simulink model "BodeConSimulink_perdidas"  (R2021b)
settings: Solver=ode23t  StartTime=0.0  StopTime=50e-3  RelTol=1e-3
values from neighbouring files (symbols this model uses):
  amp_bode = amp_bode*0.5    (= 0.003)    [BodeMatlab.m]
  Duty = 0.5    [BodeMatlab.m]
  freq_bode = frec(k)    [BodeMatlab.m]
  sampling = 0.1e-6    (= 1e-07)    [BodeMatlab.m]
libraries: fl_lib x8, nesl_utility x3
settings Model: Creator=PC  LastModifiedBy=PC

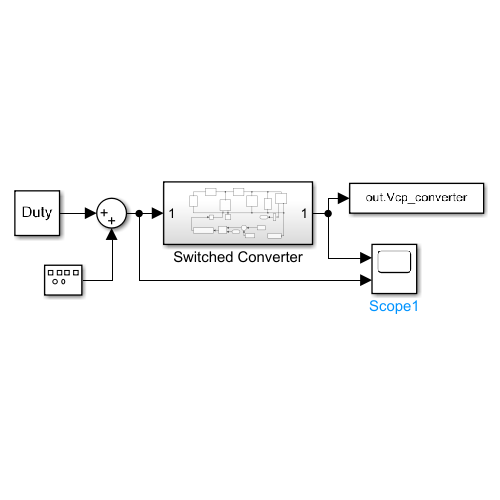
[thumbnail: Simulink's stored preview of the top-level diagram]
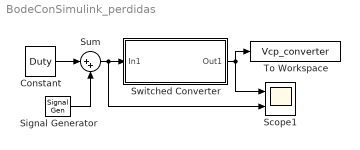
== system BodeConSimulink_perdidas ==
  " Switched Converter " : Subsystem
  Constant : Constant  Value=Duty  VectorParams1D=off  SampleTime=sampling
  Scope1 : Scope  NumInputPorts=2
  Signal Generator : SignalGenerator  Amplitude=amp_bode  Frequency=freq_bode
  Sum : Sum  Inputs=|++
  To Workspace : ToWorkspace  VariableName=Vcp_converter  SaveFormat=Structure With Time  SampleTime=-1
  wires:
  " Switched Converter "/1(Out1) -> Scope1/1, To Workspace/1
  Constant/1 -> Sum/1
  Sum/1 -> Scope1/2, " Switched Converter "/1(In1)
  Signal Generator/1 -> Sum/2

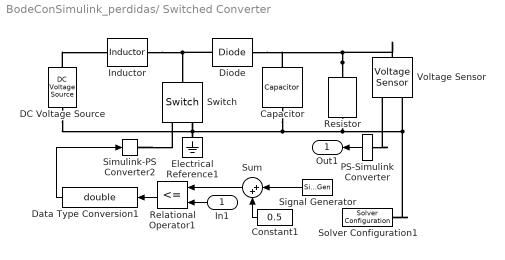
== system BodeConSimulink_perdidas/ Switched Converter  ==
  In1 : Inport
  Capacitor : fl_lib/Electrical/Electrical Elements/Capacitor  c=23 uF  r=20e-3 Ohm  g=0 1/Ohm  i_specify=off  i_priority=None  i=0 A  i_nominal_specify=off  i_nominal_unit=A  i_nominal_value=1  v_specify=off  v_priority=None  v=0 V  v_nominal_specify=off  v_nominal_unit=V  v_nominal_value=1  vc_specify=off  vc_priority=High  vc=0 V  vc_nominal_specify=off  vc_nominal_unit=V  vc_nominal_value=1
  Constant1 : Constant  Value=0.5  SampleTime=sampling
  DC Voltage Source : fl_lib/Electrical/Electrical Sources/DC Voltage Source  v0=12 V
  Data Type Conversion1 : DataTypeConversion  OutDataTypeStr=double
  Diode : fl_lib/Electrical/Electrical Elements/Diode  Vf=1.5 V  Ron=0.72 Ohm  Goff=1e-8 1/Ohm  i_specify=off  i_priority=None  i=0 A  i_nominal_specify=off  i_nominal_unit=A  i_nominal_value=1  v_specify=off  v_priority=None  v=0 V  v_nominal_specify=off  v_nominal_unit=V  v_nominal_value=1
  Electrical Reference1 : fl_lib/Electrical/Electrical Elements/Electrical Reference
  Inductor : fl_lib/Electrical/Electrical Elements/Inductor  l=130.2 uH  r=130e-3 Ohm  g=0 1/Ohm  i_specify=off  i_priority=None  i=0 A  i_nominal_specify=off  i_nominal_unit=A  i_nominal_value=1  v_specify=off  v_priority=None  v=0 V  v_nominal_specify=off  v_nominal_unit=V  v_nominal_value=1  i_L_specify=off  i_L_priority=High  i_L=0 A  i_L_nominal_specify=off  i_L_nominal_unit=A  i_L_nominal_value=1
  PS-Simulink Converter : nesl_utility/PS-Simulink Converter  PhysicalDomain=network_engine_domain  SubClassName=ps_output  LeftPortType=input  RightPortType=output  PseudoPeriodic=off  Frequencies=[]  Unit=inherit  AffineConversion=off
      settings: SourceProductBaseCode=PW,SS
  Relational Operator1 : RelationalOperator  Operator=<=  OutDataTypeStr=boolean  RndMeth=Simplest
  Resistor : fl_lib/Electrical/Electrical Elements/Resistor  R=50 Ohm  i_specify=off  i_priority=None  i=0 A  i_nominal_specify=off  i_nominal_unit=A  i_nominal_value=1  v_specify=off  v_priority=None  v=0 V  v_nominal_specify=off  v_nominal_unit=V  v_nominal_value=1
  Signal Generator : SignalGenerator  WaveForm=sawtooth  Amplitude=0.5  Frequency=50e3
  Simulink-PS Converter2 : nesl_utility/Simulink-PS Converter  PhysicalDomain=network_engine_domain  SubClassName=ps_input  LeftPortType=input  RightPortType=output  PseudoPeriodic=off  Frequencies=[]  NoiseDistribution=none  NoiseParameters=[]  Unit=V  AffineConversion=off  FilteringAndDerivatives=provide  SimscapeFilterOrder=1  InputFilterTimeConstant=0.001  UdotUserProvided=0
      settings: SourceProductBaseCode=PW,SS
  Solver Configuration1 : nesl_utility/Solver Configuration  PhysicalDomain=network_engine_domain  SubClassName=solver  LeftPortType=input  RightPortType=generic  Tones=[]  Harmonics=[]  SimulateNoise=off  Profile=off  UseLocalSampling=off  EnableSwitchedLinearOptims=on  FrequencyDomain=off  UseCCode=off  RelTol=0.001  AbsTol=1e-06  MinStep=1e-09  ToWorkspace=off  RevertToSquareIcSolve=off  NumHomotopyIterations=100  PhasorMode=off  PhasorModeNumHarmonics=1  DoDC=off  ResidualTolerance=1e-09  UseLocalSolver=off  LocalSolverChoice=NE_BACKWARD_EULER_ADVANCER  LocalSolverSampleTime=0.001  DoFixedCost=off  MaxNonlinIter=3  MaxModeIter=2  ComputeImpulses=off  ImpulseIterations=2  LinearAlgebra=auto  EquationFormulation=NE_TIME_EF  DelaysMemoryBudget=1024  AutomaticFiltering=on  FilteringTimeConstant=sampling  PartitionStorageMethod=AS_NEEDED  PartitionMemoryBudget=1024  PartitionMethod=ROBUST
      settings: SourceProductBaseCode=PW,SS
  Sum : Sum  Inputs=|++
  Switch : fl_lib/Electrical/Electrical Elements/Switch  R_closed=77e-3 Ohm  G_open=1e-8 1/Ohm  Threshold=0.5  i_specify=off  i_priority=None  i=0 A  i_nominal_specify=off  i_nominal_unit=A  i_nominal_value=1  v_specify=off  v_priority=None  v=0 V  v_nominal_specify=off  v_nominal_unit=V  v_nominal_value=1
  Voltage Sensor : fl_lib/Electrical/Electrical Sensors/Voltage Sensor
  Out1 : Outport
  wires:
  Signal Generator/1 -> Sum/1
  Relational Operator1/1 -> Data Type Conversion1/1
  In1/1 -> Relational Operator1/2
  Sum/1 -> Relational Operator1/1
  Constant1/1 -> Sum/2
  Data Type Conversion1/1 -> Simulink-PS Converter2/1
  PS-Simulink Converter/1 -> Out1/1
  connections:
  Electrical Reference1/LConn1 -- Switch/RConn2 -- Resistor/RConn1 -- Voltage Sensor/RConn2 -- Solver Configuration1/RConn1 -- Capacitor/RConn1 -- DC Voltage Source/RConn1
  Diode/LConn1 -- Inductor/RConn1 -- Switch/LConn1
  DC Voltage Source/LConn1 -- Inductor/LConn1
  Resistor/LConn1 -- Voltage Sensor/LConn1 -- Diode/RConn1 -- Capacitor/LConn1
  Simulink-PS Converter2/RConn1 -- Switch/RConn1
  PS-Simulink Converter/LConn1 -- Voltage Sensor/RConn1
